simulink model "BEV_Laengsdynamikmodell_v2"  (R2023b)
settings: configuration reference "SharedConfig" (kept outside this file)
undefined symbols (not defined in the file): acc_cycle_flag, Analyse, battery, battery_builder_rtmsupport, config_battery, config_gearbox, config_Inverter, config_motor, config_vehicle, GB, gcbh, gearbox_map, k_FW, ModuleAssembly1, ModuleType1, motormap, motormap2
libraries: powerlib x37, nesl_utility x18, GD_Batterymodel_NSGAII_1_lib x12, BatteryProtection x9, fl_lib x7, dspstat3 x4, simulink x3, eePmsmCurrentReferenceGen x2, spsControlledCurrentSourceLib x2, spsVoltageMeasurementLib x2, batt_lib x1, BatteryBalancing x1
(part 5 of 6)

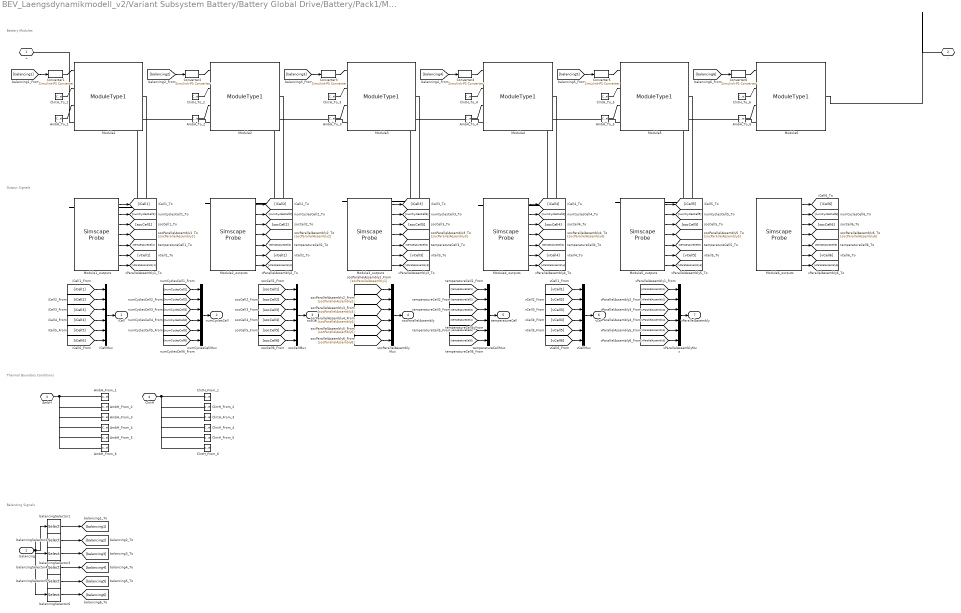
== system BEV_Laengsdynamikmodell_v2/Variant Subsystem Battery/Battery Global Drive/Battery/Pack1/ModuleAssembly2 ==
  note: Battery Modules
  note: Output Signals
  note: Thermal Boundary Conditions
  note: Balancing Signals
  balancing : Inport  PortDimensions=108
  AmbH_From_1 : ConnectionLabel  Label=ambH_1
  AmbH_From_2 : ConnectionLabel  Label=ambH_2
  AmbH_From_3 : ConnectionLabel  Label=ambH_3
  AmbH_From_4 : ConnectionLabel  Label=ambH_4
  AmbH_From_5 : ConnectionLabel  Label=ambH_5
  AmbH_From_6 : ConnectionLabel  Label=ambH_6
  AmbH_To_1 : ConnectionLabel  Label=ambH_1
  AmbH_To_2 : ConnectionLabel  Label=ambH_2
  AmbH_To_3 : ConnectionLabel  Label=ambH_3
  AmbH_To_4 : ConnectionLabel  Label=ambH_4
  AmbH_To_5 : ConnectionLabel  Label=ambH_5
  AmbH_To_6 : ConnectionLabel  Label=ambH_6
  ClntH_From_1 : ConnectionLabel  Label=clntH_1
  ClntH_From_2 : ConnectionLabel  Label=clntH_2
  ClntH_From_3 : ConnectionLabel  Label=clntH_3
  ClntH_From_4 : ConnectionLabel  Label=clntH_4
  ClntH_From_5 : ConnectionLabel  Label=clntH_5
  ClntH_From_6 : ConnectionLabel  Label=clntH_6
  ClntH_To_1 : ConnectionLabel  Label=clntH_1
  ClntH_To_2 : ConnectionLabel  Label=clntH_2
  ClntH_To_3 : ConnectionLabel  Label=clntH_3
  ClntH_To_4 : ConnectionLabel  Label=clntH_4
  ClntH_To_5 : ConnectionLabel  Label=clntH_5
  ClntH_To_6 : ConnectionLabel  Label=clntH_6
  Converter{1..6} (6 alike) : nesl_utility/Simulink-PS Converter  PhysicalDomain=network_engine_domain  SubClassName=ps_input  LeftPortType=input  RightPortType=output  PseudoPeriodic=off  Frequencies=[]  NoiseDistribution=none  NoiseParameters=[]  Unit=1  AffineConversion=off  FilteringAndDerivatives=provide  SimscapeFilterOrder=1  InputFilterTimeConstant=0.001  UdotUserProvided=0
  Module1 : GD_Batterymodel_NSGAII_1_lib/Modules/ModuleType1  SOC_vecCell=ModuleType1.SOC_vecCell  T_vecCell=ModuleType1.T_vecCell K  V0_matCell=ModuleType1.V0_matCell V  V_rangeCell=ModuleType1.V_rangeCell V  R0_matCell=ModuleType1.R0_matCell Ohm  AHCell=ModuleType1.AHCell A*hr  extrapolation_optionCell=simscape.enum.extrapolation.nearest  R1_matCell=ModuleType1.R1_matCell Ohm  tau1_matCell=ModuleType1.tau1_matCell s  R2_matCell=ModuleType1.R2_matCell Ohm  tau2_matCell=ModuleType1.tau2_matCell s  thermal_massCell=ModuleType1.thermal_massCell J/K  CoolantResistance=ModuleType1.CoolantResistance K/W  AmbientResistance=ModuleType1.AmbientResistance K/W  CellBalancingClosedResistance=ModuleType1.CellBalancingClosedResistance Ohm  CellBalancingOpenConductance=ModuleType1.CellBalancingOpenConductance 1/Ohm  CellBalancingThreshold=ModuleType1.CellBalancingThreshold  CellBalancingResistance=ModuleType1.CellBalancingResistance Ohm  P=1  S=18  iCell_specify=on  iCell_priority=None  iCell=ModuleAssembly2.Module1.iCell A  iCell_nominal_specify=off  iCell_nominal_unit=A  iCell_nominal_value=1  vCell_specify=on  vCell_priority=None  vCell=ModuleAssembly2.Module1.vCell V  vCell_nominal_specify=off  vCell_nominal_unit=V  vCell_nominal_value=1  socCell_specify=on  socCell_priority=High  socCell=ModuleAssembly2.Module1.socCell  socCell_nominal_specify=off  socCell_nominal_unit=1  socCell_nominal_value=1  numCyclesCell_specify=on  numCyclesCell_priority=High  numCyclesCell=ModuleAssembly2.Module1.numCyclesCell  numCyclesCell_nominal_specify=off  numCyclesCell_nominal_unit=1  numCyclesCell_nominal_value=1  temperatureCell_specify=on  temperatureCell_priority=High  temperatureCell=ModuleAssembly2.Module1.temperatureCell K  temperatureCell_nominal_specify=off  temperatureCell_nominal_unit=K  temperatureCell_nominal_value=1  vParallelAssembly_specify=on  vParallelAssembly_priority=None  vParallelAssembly=ModuleAssembly2.Module1.vParallelAssembly V  vParallelAssembly_nominal_specify=off  vParallelAssembly_nominal_unit=V  vParallelAssembly_nominal_value=1  socParallelAssembly_specify=on  socParallelAssembly_priority=None  socParallelAssembly=ModuleAssembly2.Module1.socParallelAssembly  socParallelAssembly_nominal_specify=off  socParallelAssembly_nominal_unit=1  socParallelAssembly_nominal_value=1
      settings: InternalSimscapePortConfiguration="{\"Bottom\":[{\"id\":\"n\",\"label\":\"-\",\"type\":\"foundation.electrical.electrical\"}],\"Left\":[{\"id\":\"enableCellBalancing\",\"label\":\"CB\",\"type\":\"input\"},{\"id\":\"ClntH\",\"label\":\"ClntH\",\"type\":\"foundation.thermal.thermal\"},{\"id\":\"AmbH\",\"label\":\"AmbH\",\"type\":\"foundation.thermal.thermal\"}],\"Right\":[],\"Top\":[{\"id\":\"p\",\"label\":\"+\",\"type\":\"foundation.electrical.electrical\"}]}"
  Module1_outputs : SimscapeProbe  BoundBlock=292794  Variables={iCell, numCyclesCell, socCell, socParallelAssembly, temperatureCell, vCell, vParallelAssembly}
  Module2 : GD_Batterymodel_NSGAII_1_lib/Modules/ModuleType1  SOC_vecCell=ModuleType1.SOC_vecCell  T_vecCell=ModuleType1.T_vecCell K  V0_matCell=ModuleType1.V0_matCell V  V_rangeCell=ModuleType1.V_rangeCell V  R0_matCell=ModuleType1.R0_matCell Ohm  AHCell=ModuleType1.AHCell A*hr  extrapolation_optionCell=simscape.enum.extrapolation.nearest  R1_matCell=ModuleType1.R1_matCell Ohm  tau1_matCell=ModuleType1.tau1_matCell s  R2_matCell=ModuleType1.R2_matCell Ohm  tau2_matCell=ModuleType1.tau2_matCell s  thermal_massCell=ModuleType1.thermal_massCell J/K  CoolantResistance=ModuleType1.CoolantResistance K/W  AmbientResistance=ModuleType1.AmbientResistance K/W  CellBalancingClosedResistance=ModuleType1.CellBalancingClosedResistance Ohm  CellBalancingOpenConductance=ModuleType1.CellBalancingOpenConductance 1/Ohm  CellBalancingThreshold=ModuleType1.CellBalancingThreshold  CellBalancingResistance=ModuleType1.CellBalancingResistance Ohm  P=1  S=18  iCell_specify=on  iCell_priority=None  iCell=ModuleAssembly2.Module2.iCell A  iCell_nominal_specify=off  iCell_nominal_unit=A  iCell_nominal_value=1  vCell_specify=on  vCell_priority=None  vCell=ModuleAssembly2.Module2.vCell V  vCell_nominal_specify=off  vCell_nominal_unit=V  vCell_nominal_value=1  socCell_specify=on  socCell_priority=High  socCell=ModuleAssembly2.Module2.socCell  socCell_nominal_specify=off  socCell_nominal_unit=1  socCell_nominal_value=1  numCyclesCell_specify=on  numCyclesCell_priority=High  numCyclesCell=ModuleAssembly2.Module2.numCyclesCell  numCyclesCell_nominal_specify=off  numCyclesCell_nominal_unit=1  numCyclesCell_nominal_value=1  temperatureCell_specify=on  temperatureCell_priority=High  temperatureCell=ModuleAssembly2.Module2.temperatureCell K  temperatureCell_nominal_specify=off  temperatureCell_nominal_unit=K  temperatureCell_nominal_value=1  vParallelAssembly_specify=on  vParallelAssembly_priority=None  vParallelAssembly=ModuleAssembly2.Module2.vParallelAssembly V  vParallelAssembly_nominal_specify=off  vParallelAssembly_nominal_unit=V  vParallelAssembly_nominal_value=1  socParallelAssembly_specify=on  socParallelAssembly_priority=None  socParallelAssembly=ModuleAssembly2.Module2.socParallelAssembly  socParallelAssembly_nominal_specify=off  socParallelAssembly_nominal_unit=1  socParallelAssembly_nominal_value=1
      settings: InternalSimscapePortConfiguration="{\"Bottom\":[{\"id\":\"n\",\"label\":\"-\",\"type\":\"foundation.electrical.electrical\"}],\"Left\":[{\"id\":\"enableCellBalancing\",\"label\":\"CB\",\"type\":\"input\"},{\"id\":\"ClntH\",\"label\":\"ClntH\",\"type\":\"foundation.thermal.thermal\"},{\"id\":\"AmbH\",\"label\":\"AmbH\",\"type\":\"foundation.thermal.thermal\"}],\"Right\":[],\"Top\":[{\"id\":\"p\",\"label\":\"+\",\"type\":\"foundation.electrical.electrical\"}]}"
  Module2_outputs : SimscapeProbe  BoundBlock=292796  Variables={iCell, numCyclesCell, socCell, socParallelAssembly, temperatureCell, vCell, vParallelAssembly}
  Module3 : GD_Batterymodel_NSGAII_1_lib/Modules/ModuleType1  SOC_vecCell=ModuleType1.SOC_vecCell  T_vecCell=ModuleType1.T_vecCell K  V0_matCell=ModuleType1.V0_matCell V  V_rangeCell=ModuleType1.V_rangeCell V  R0_matCell=ModuleType1.R0_matCell Ohm  AHCell=ModuleType1.AHCell A*hr  extrapolation_optionCell=simscape.enum.extrapolation.nearest  R1_matCell=ModuleType1.R1_matCell Ohm  tau1_matCell=ModuleType1.tau1_matCell s  R2_matCell=ModuleType1.R2_matCell Ohm  tau2_matCell=ModuleType1.tau2_matCell s  thermal_massCell=ModuleType1.thermal_massCell J/K  CoolantResistance=ModuleType1.CoolantResistance K/W  AmbientResistance=ModuleType1.AmbientResistance K/W  CellBalancingClosedResistance=ModuleType1.CellBalancingClosedResistance Ohm  CellBalancingOpenConductance=ModuleType1.CellBalancingOpenConductance 1/Ohm  CellBalancingThreshold=ModuleType1.CellBalancingThreshold  CellBalancingResistance=ModuleType1.CellBalancingResistance Ohm  P=1  S=18  iCell_specify=on  iCell_priority=None  iCell=ModuleAssembly2.Module3.iCell A  iCell_nominal_specify=off  iCell_nominal_unit=A  iCell_nominal_value=1  vCell_specify=on  vCell_priority=None  vCell=ModuleAssembly2.Module3.vCell V  vCell_nominal_specify=off  vCell_nominal_unit=V  vCell_nominal_value=1  socCell_specify=on  socCell_priority=High  socCell=ModuleAssembly2.Module3.socCell  socCell_nominal_specify=off  socCell_nominal_unit=1  socCell_nominal_value=1  numCyclesCell_specify=on  numCyclesCell_priority=High  numCyclesCell=ModuleAssembly2.Module3.numCyclesCell  numCyclesCell_nominal_specify=off  numCyclesCell_nominal_unit=1  numCyclesCell_nominal_value=1  temperatureCell_specify=on  temperatureCell_priority=High  temperatureCell=ModuleAssembly2.Module3.temperatureCell K  temperatureCell_nominal_specify=off  temperatureCell_nominal_unit=K  temperatureCell_nominal_value=1  vParallelAssembly_specify=on  vParallelAssembly_priority=None  vParallelAssembly=ModuleAssembly2.Module3.vParallelAssembly V  vParallelAssembly_nominal_specify=off  vParallelAssembly_nominal_unit=V  vParallelAssembly_nominal_value=1  socParallelAssembly_specify=on  socParallelAssembly_priority=None  socParallelAssembly=ModuleAssembly2.Module3.socParallelAssembly  socParallelAssembly_nominal_specify=off  socParallelAssembly_nominal_unit=1  socParallelAssembly_nominal_value=1
      settings: InternalSimscapePortConfiguration="{\"Bottom\":[{\"id\":\"n\",\"label\":\"-\",\"type\":\"foundation.electrical.electrical\"}],\"Left\":[{\"id\":\"enableCellBalancing\",\"label\":\"CB\",\"type\":\"input\"},{\"id\":\"ClntH\",\"label\":\"ClntH\",\"type\":\"foundation.thermal.thermal\"},{\"id\":\"AmbH\",\"label\":\"AmbH\",\"type\":\"foundation.thermal.thermal\"}],\"Right\":[],\"Top\":[{\"id\":\"p\",\"label\":\"+\",\"type\":\"foundation.electrical.electrical\"}]}"
  Module3_outputs : SimscapeProbe  BoundBlock=292798  Variables={iCell, numCyclesCell, socCell, socParallelAssembly, temperatureCell, vCell, vParallelAssembly}
  Module4 : GD_Batterymodel_NSGAII_1_lib/Modules/ModuleType1  SOC_vecCell=ModuleType1.SOC_vecCell  T_vecCell=ModuleType1.T_vecCell K  V0_matCell=ModuleType1.V0_matCell V  V_rangeCell=ModuleType1.V_rangeCell V  R0_matCell=ModuleType1.R0_matCell Ohm  AHCell=ModuleType1.AHCell A*hr  extrapolation_optionCell=simscape.enum.extrapolation.nearest  R1_matCell=ModuleType1.R1_matCell Ohm  tau1_matCell=ModuleType1.tau1_matCell s  R2_matCell=ModuleType1.R2_matCell Ohm  tau2_matCell=ModuleType1.tau2_matCell s  thermal_massCell=ModuleType1.thermal_massCell J/K  CoolantResistance=ModuleType1.CoolantResistance K/W  AmbientResistance=ModuleType1.AmbientResistance K/W  CellBalancingClosedResistance=ModuleType1.CellBalancingClosedResistance Ohm  CellBalancingOpenConductance=ModuleType1.CellBalancingOpenConductance 1/Ohm  CellBalancingThreshold=ModuleType1.CellBalancingThreshold  CellBalancingResistance=ModuleType1.CellBalancingResistance Ohm  P=1  S=18  iCell_specify=on  iCell_priority=None  iCell=ModuleAssembly2.Module4.iCell A  iCell_nominal_specify=off  iCell_nominal_unit=A  iCell_nominal_value=1  vCell_specify=on  vCell_priority=None  vCell=ModuleAssembly2.Module4.vCell V  vCell_nominal_specify=off  vCell_nominal_unit=V  vCell_nominal_value=1  socCell_specify=on  socCell_priority=High  socCell=ModuleAssembly2.Module4.socCell  socCell_nominal_specify=off  socCell_nominal_unit=1  socCell_nominal_value=1  numCyclesCell_specify=on  numCyclesCell_priority=High  numCyclesCell=ModuleAssembly2.Module4.numCyclesCell  numCyclesCell_nominal_specify=off  numCyclesCell_nominal_unit=1  numCyclesCell_nominal_value=1  temperatureCell_specify=on  temperatureCell_priority=High  temperatureCell=ModuleAssembly2.Module4.temperatureCell K  temperatureCell_nominal_specify=off  temperatureCell_nominal_unit=K  temperatureCell_nominal_value=1  vParallelAssembly_specify=on  vParallelAssembly_priority=None  vParallelAssembly=ModuleAssembly2.Module4.vParallelAssembly V  vParallelAssembly_nominal_specify=off  vParallelAssembly_nominal_unit=V  vParallelAssembly_nominal_value=1  socParallelAssembly_specify=on  socParallelAssembly_priority=None  socParallelAssembly=ModuleAssembly2.Module4.socParallelAssembly  socParallelAssembly_nominal_specify=off  socParallelAssembly_nominal_unit=1  socParallelAssembly_nominal_value=1
      settings: InternalSimscapePortConfiguration="{\"Bottom\":[{\"id\":\"n\",\"label\":\"-\",\"type\":\"foundation.electrical.electrical\"}],\"Left\":[{\"id\":\"enableCellBalancing\",\"label\":\"CB\",\"type\":\"input\"},{\"id\":\"ClntH\",\"label\":\"ClntH\",\"type\":\"foundation.thermal.thermal\"},{\"id\":\"AmbH\",\"label\":\"AmbH\",\"type\":\"foundation.thermal.thermal\"}],\"Right\":[],\"Top\":[{\"id\":\"p\",\"label\":\"+\",\"type\":\"foundation.electrical.electrical\"}]}"
  Module4_outputs : SimscapeProbe  BoundBlock=292800  Variables={iCell, numCyclesCell, socCell, socParallelAssembly, temperatureCell, vCell, vParallelAssembly}
  Module5 : GD_Batterymodel_NSGAII_1_lib/Modules/ModuleType1  SOC_vecCell=ModuleType1.SOC_vecCell  T_vecCell=ModuleType1.T_vecCell K  V0_matCell=ModuleType1.V0_matCell V  V_rangeCell=ModuleType1.V_rangeCell V  R0_matCell=ModuleType1.R0_matCell Ohm  AHCell=ModuleType1.AHCell A*hr  extrapolation_optionCell=simscape.enum.extrapolation.nearest  R1_matCell=ModuleType1.R1_matCell Ohm  tau1_matCell=ModuleType1.tau1_matCell s  R2_matCell=ModuleType1.R2_matCell Ohm  tau2_matCell=ModuleType1.tau2_matCell s  thermal_massCell=ModuleType1.thermal_massCell J/K  CoolantResistance=ModuleType1.CoolantResistance K/W  AmbientResistance=ModuleType1.AmbientResistance K/W  CellBalancingClosedResistance=ModuleType1.CellBalancingClosedResistance Ohm  CellBalancingOpenConductance=ModuleType1.CellBalancingOpenConductance 1/Ohm  CellBalancingThreshold=ModuleType1.CellBalancingThreshold  CellBalancingResistance=ModuleType1.CellBalancingResistance Ohm  P=1  S=18  iCell_specify=on  iCell_priority=None  iCell=ModuleAssembly2.Module5.iCell A  iCell_nominal_specify=off  iCell_nominal_unit=A  iCell_nominal_value=1  vCell_specify=on  vCell_priority=None  vCell=ModuleAssembly2.Module5.vCell V  vCell_nominal_specify=off  vCell_nominal_unit=V  vCell_nominal_value=1  socCell_specify=on  socCell_priority=High  socCell=ModuleAssembly2.Module5.socCell  socCell_nominal_specify=off  socCell_nominal_unit=1  socCell_nominal_value=1  numCyclesCell_specify=on  numCyclesCell_priority=High  numCyclesCell=ModuleAssembly2.Module5.numCyclesCell  numCyclesCell_nominal_specify=off  numCyclesCell_nominal_unit=1  numCyclesCell_nominal_value=1  temperatureCell_specify=on  temperatureCell_priority=High  temperatureCell=ModuleAssembly2.Module5.temperatureCell K  temperatureCell_nominal_specify=off  temperatureCell_nominal_unit=K  temperatureCell_nominal_value=1  vParallelAssembly_specify=on  vParallelAssembly_priority=None  vParallelAssembly=ModuleAssembly2.Module5.vParallelAssembly V  vParallelAssembly_nominal_specify=off  vParallelAssembly_nominal_unit=V  vParallelAssembly_nominal_value=1  socParallelAssembly_specify=on  socParallelAssembly_priority=None  socParallelAssembly=ModuleAssembly2.Module5.socParallelAssembly  socParallelAssembly_nominal_specify=off  socParallelAssembly_nominal_unit=1  socParallelAssembly_nominal_value=1
      settings: InternalSimscapePortConfiguration="{\"Bottom\":[{\"id\":\"n\",\"label\":\"-\",\"type\":\"foundation.electrical.electrical\"}],\"Left\":[{\"id\":\"enableCellBalancing\",\"label\":\"CB\",\"type\":\"input\"},{\"id\":\"ClntH\",\"label\":\"ClntH\",\"type\":\"foundation.thermal.thermal\"},{\"id\":\"AmbH\",\"label\":\"AmbH\",\"type\":\"foundation.thermal.thermal\"}],\"Right\":[],\"Top\":[{\"id\":\"p\",\"label\":\"+\",\"type\":\"foundation.electrical.electrical\"}]}"
  Module5_outputs : SimscapeProbe  BoundBlock=292802  Variables={iCell, numCyclesCell, socCell, socParallelAssembly, temperatureCell, vCell, vParallelAssembly}
  Module6 : GD_Batterymodel_NSGAII_1_lib/Modules/ModuleType1  SOC_vecCell=ModuleType1.SOC_vecCell  T_vecCell=ModuleType1.T_vecCell K  V0_matCell=ModuleType1.V0_matCell V  V_rangeCell=ModuleType1.V_rangeCell V  R0_matCell=ModuleType1.R0_matCell Ohm  AHCell=ModuleType1.AHCell A*hr  extrapolation_optionCell=simscape.enum.extrapolation.nearest  R1_matCell=ModuleType1.R1_matCell Ohm  tau1_matCell=ModuleType1.tau1_matCell s  R2_matCell=ModuleType1.R2_matCell Ohm  tau2_matCell=ModuleType1.tau2_matCell s  thermal_massCell=ModuleType1.thermal_massCell J/K  CoolantResistance=ModuleType1.CoolantResistance K/W  AmbientResistance=ModuleType1.AmbientResistance K/W  CellBalancingClosedResistance=ModuleType1.CellBalancingClosedResistance Ohm  CellBalancingOpenConductance=ModuleType1.CellBalancingOpenConductance 1/Ohm  CellBalancingThreshold=ModuleType1.CellBalancingThreshold  CellBalancingResistance=ModuleType1.CellBalancingResistance Ohm  P=1  S=18  iCell_specify=on  iCell_priority=None  iCell=ModuleAssembly2.Module6.iCell A  iCell_nominal_specify=off  iCell_nominal_unit=A  iCell_nominal_value=1  vCell_specify=on  vCell_priority=None  vCell=ModuleAssembly2.Module6.vCell V  vCell_nominal_specify=off  vCell_nominal_unit=V  vCell_nominal_value=1  socCell_specify=on  socCell_priority=High  socCell=ModuleAssembly2.Module6.socCell  socCell_nominal_specify=off  socCell_nominal_unit=1  socCell_nominal_value=1  numCyclesCell_specify=on  numCyclesCell_priority=High  numCyclesCell=ModuleAssembly2.Module6.numCyclesCell  numCyclesCell_nominal_specify=off  numCyclesCell_nominal_unit=1  numCyclesCell_nominal_value=1  temperatureCell_specify=on  temperatureCell_priority=High  temperatureCell=ModuleAssembly2.Module6.temperatureCell K  temperatureCell_nominal_specify=off  temperatureCell_nominal_unit=K  temperatureCell_nominal_value=1  vParallelAssembly_specify=on  vParallelAssembly_priority=None  vParallelAssembly=ModuleAssembly2.Module6.vParallelAssembly V  vParallelAssembly_nominal_specify=off  vParallelAssembly_nominal_unit=V  vParallelAssembly_nominal_value=1  socParallelAssembly_specify=on  socParallelAssembly_priority=None  socParallelAssembly=ModuleAssembly2.Module6.socParallelAssembly  socParallelAssembly_nominal_specify=off  socParallelAssembly_nominal_unit=1  socParallelAssembly_nominal_value=1
      settings: InternalSimscapePortConfiguration="{\"Bottom\":[{\"id\":\"n\",\"label\":\"-\",\"type\":\"foundation.electrical.electrical\"}],\"Left\":[{\"id\":\"enableCellBalancing\",\"label\":\"CB\",\"type\":\"input\"},{\"id\":\"ClntH\",\"label\":\"ClntH\",\"type\":\"foundation.thermal.thermal\"},{\"id\":\"AmbH\",\"label\":\"AmbH\",\"type\":\"foundation.thermal.thermal\"}],\"Right\":[],\"Top\":[{\"id\":\"p\",\"label\":\"+\",\"type\":\"foundation.electrical.electrical\"}]}"
  Module6_outputs : SimscapeProbe  BoundBlock=292804  Variables={iCell, numCyclesCell, socCell, socParallelAssembly, temperatureCell, vCell, vParallelAssembly}
  balancingSelector1 : Selector  InputPortWidth=108  IndexOptions=Index vector (dialog)  Indices="[1   2   3   4   5   6   7   8   9  10  11  12  13  14  15  16  17  18]"  OutputSizes=1
  balancingSelector2 : Selector  InputPortWidth=108  IndexOptions=Index vector (dialog)  Indices="[19  20  21  22  23  24  25  26  27  28  29  30  31  32  33  34  35  36]"  OutputSizes=1
  balancingSelector3 : Selector  InputPortWidth=108  IndexOptions=Index vector (dialog)  Indices="[37  38  39  40  41  42  43  44  45  46  47  48  49  50  51  52  53  54]"  OutputSizes=1
  balancingSelector4 : Selector  InputPortWidth=108  IndexOptions=Index vector (dialog)  Indices="[55  56  57  58  59  60  61  62  63  64  65  66  67  68  69  70  71  72]"  OutputSizes=1
  balancingSelector5 : Selector  InputPortWidth=108  IndexOptions=Index vector (dialog)  Indices="[73  74  75  76  77  78  79  80  81  82  83  84  85  86  87  88  89  90]"  OutputSizes=1
  balancingSelector6 : Selector  InputPortWidth=108  IndexOptions=Index vector (dialog)  Indices="[91   92   93   94   95   96   97   98   99  100  101  102  103  104  105  106  107  108]"  OutputSizes=1
  iCellMux : Mux  Inputs=6
  numCyclesCellMux : Mux  Inputs=6
  socCellMux : Mux  Inputs=6
  socParallelAssemblyMux : Mux  Inputs=6
  temperatureCellMux : Mux  Inputs=6
  vCellMux : Mux  Inputs=6
  vParallelAssemblyMux : Mux  Inputs=6
  + : PMIOPort  Side=Left
  - : PMIOPort  Port=2  Side=Right
  AmbH : PMIOPort  Port=3  Side=Right  ConnectionType=Connection: foundation.thermal.thermal
  ClntH : PMIOPort  Port=4  Side=Right  ConnectionType=Connection: foundation.thermal.thermal
  iCell : Outport
  numCyclesCell : Outport  Port=2
  socCell : Outport  Port=3
  socParallelAssembly : Outport  Port=4
  temperatureCell : Outport  Port=5
  vCell : Outport  Port=6
  vParallelAssembly : Outport  Port=7
  wires:
  Module1_outputs/1 -> [iCell1]
  iCellMux/1 -> iCell/1
  [iCell1] -> iCellMux/1
  Module1_outputs/2 -> [numCyclesCell1]
  numCyclesCellMux/1 -> numCyclesCell/1
  [numCyclesCell1] -> numCyclesCellMux/1
  Module1_outputs/3 -> [socCell1]
  socCellMux/1 -> socCell/1
  [socCell1] -> socCellMux/1
  Module1_outputs/4 -> [socParallelAssembly1]
  socParallelAssemblyMux/1 -> socParallelAssembly/1
  [socParallelAssembly1] -> socParallelAssemblyMux/1
  Module1_outputs/5 -> [temperatureCell1]
  temperatureCellMux/1 -> temperatureCell/1
  [temperatureCell1] -> temperatureCellMux/1
  Module1_outputs/6 -> [vCell1]
  vCellMux/1 -> vCell/1
  [vCell1] -> vCellMux/1
  Module1_outputs/7 -> [vParallelAssembly1]
  vParallelAssemblyMux/1 -> vParallelAssembly/1
  [vParallelAssembly1] -> vParallelAssemblyMux/1
  Module2_outputs/1 -> [iCell2]
  [iCell2] -> iCellMux/2
  Module2_outputs/2 -> [numCyclesCell2]
  [numCyclesCell2] -> numCyclesCellMux/2
  Module2_outputs/3 -> [socCell2]
  [socCell2] -> socCellMux/2
  Module2_outputs/4 -> [socParallelAssembly2]
  [socParallelAssembly2] -> socParallelAssemblyMux/2
  Module2_outputs/5 -> [temperatureCell2]
  [temperatureCell2] -> temperatureCellMux/2
  Module2_outputs/6 -> [vCell2]
  [vCell2] -> vCellMux/2
  Module2_outputs/7 -> [vParallelAssembly2]
  [vParallelAssembly2] -> vParallelAssemblyMux/2
  Module3_outputs/1 -> [iCell3]
  [iCell3] -> iCellMux/3
  Module3_outputs/2 -> [numCyclesCell3]
  [numCyclesCell3] -> numCyclesCellMux/3
  Module3_outputs/3 -> [socCell3]
  [socCell3] -> socCellMux/3
  Module3_outputs/4 -> [socParallelAssembly3]
  [socParallelAssembly3] -> socParallelAssemblyMux/3
  Module3_outputs/5 -> [temperatureCell3]
  [temperatureCell3] -> temperatureCellMux/3
  Module3_outputs/6 -> [vCell3]
  [vCell3] -> vCellMux/3
  Module3_outputs/7 -> [vParallelAssembly3]
  [vParallelAssembly3] -> vParallelAssemblyMux/3
  Module4_outputs/1 -> [iCell4]
  [iCell4] -> iCellMux/4
  Module4_outputs/2 -> [numCyclesCell4]
  [numCyclesCell4] -> numCyclesCellMux/4
  Module4_outputs/3 -> [socCell4]
  [socCell4] -> socCellMux/4
  Module4_outputs/4 -> [socParallelAssembly4]
  [socParallelAssembly4] -> socParallelAssemblyMux/4
  Module4_outputs/5 -> [temperatureCell4]
  [temperatureCell4] -> temperatureCellMux/4
  Module4_outputs/6 -> [vCell4]
  [vCell4] -> vCellMux/4
  Module4_outputs/7 -> [vParallelAssembly4]
  [vParallelAssembly4] -> vParallelAssemblyMux/4
  Module5_outputs/1 -> [iCell5]
  [iCell5] -> iCellMux/5
  Module5_outputs/2 -> [numCyclesCell5]
  [numCyclesCell5] -> numCyclesCellMux/5
  Module5_outputs/3 -> [socCell5]
  [socCell5] -> socCellMux/5
  Module5_outputs/4 -> [socParallelAssembly5]
  [socParallelAssembly5] -> socParallelAssemblyMux/5
  Module5_outputs/5 -> [temperatureCell5]
  [temperatureCell5] -> temperatureCellMux/5
  Module5_outputs/6 -> [vCell5]
  [vCell5] -> vCellMux/5
  Module5_outputs/7 -> [vParallelAssembly5]
  [vParallelAssembly5] -> vParallelAssemblyMux/5
  Module6_outputs/1 -> [iCell6]
  [iCell6] -> iCellMux/6
  Module6_outputs/2 -> [numCyclesCell6]
  [numCyclesCell6] -> numCyclesCellMux/6
  Module6_outputs/3 -> [socCell6]
  [socCell6] -> socCellMux/6
  Module6_outputs/4 -> [socParallelAssembly6]
  [socParallelAssembly6] -> socParallelAssemblyMux/6
  Module6_outputs/5 -> [temperatureCell6]
  [temperatureCell6] -> temperatureCellMux/6
  Module6_outputs/6 -> [vCell6]
  [vCell6] -> vCellMux/6
  Module6_outputs/7 -> [vParallelAssembly6]
  [vParallelAssembly6] -> vParallelAssemblyMux/6
  [balancing1] -> Converter1/1
  balancing/1 -> balancingSelector1/1, balancingSelector2/1, balancingSelector3/1, balancingSelector4/1, balancingSelector5/1, balancingSelector6/1
  balancingSelector1/1 -> [balancing1]
  [balancing2] -> Converter2/1
  balancingSelector2/1 -> [balancing2]
  [balancing3] -> Converter3/1
  balancingSelector3/1 -> [balancing3]
  [balancing4] -> Converter4/1
  balancingSelector4/1 -> [balancing4]
  [balancing5] -> Converter5/1
  balancingSelector5/1 -> [balancing5]
  [balancing6] -> Converter6/1
  balancingSelector6/1 -> [balancing6]
  connections:
  Module2/LConn4 -- Module1/RConn1
  Module3/LConn4 -- Module2/RConn1
  Module4/LConn4 -- Module3/RConn1
  Module5/LConn4 -- Module4/RConn1
  Module6/LConn4 -- Module5/RConn1
  Module1/LConn4 -- +/RConn1
  Module6/RConn1 -- -/RConn1
  AmbH_To_1/LConn1 -- Module1/LConn3
  AmbH_From_1/LConn1 -- AmbH_From_2/LConn1 -- AmbH_From_3/LConn1 -- AmbH_From_4/LConn1 -- AmbH_From_5/LConn1 -- AmbH/RConn1 -- AmbH_From_6/LConn1
  AmbH_To_2/LConn1 -- Module2/LConn3
  AmbH_To_3/LConn1 -- Module3/LConn3
  AmbH_To_4/LConn1 -- Module4/LConn3
  AmbH_To_5/LConn1 -- Module5/LConn3
  AmbH_To_6/LConn1 -- Module6/LConn3
  ClntH_To_1/LConn1 -- Module1/LConn2
  ClntH_From_1/LConn1 -- ClntH_From_2/LConn1 -- ClntH_From_3/LConn1 -- ClntH_From_4/LConn1 -- ClntH_From_5/LConn1 -- ClntH/RConn1 -- ClntH_From_6/LConn1
  ClntH_To_2/LConn1 -- Module2/LConn2
  ClntH_To_3/LConn1 -- Module3/LConn2
  ClntH_To_4/LConn1 -- Module4/LConn2
  ClntH_To_5/LConn1 -- Module5/LConn2
  ClntH_To_6/LConn1 -- Module6/LConn2
  Converter1/RConn1 -- Module1/LConn1
  Converter2/RConn1 -- Module2/LConn1
  Converter3/RConn1 -- Module3/LConn1
  Converter4/RConn1 -- Module4/LConn1
  Converter5/RConn1 -- Module5/LConn1
  Converter6/RConn1 -- Module6/LConn1

== system BEV_Laengsdynamikmodell_v2/Variant Subsystem Gearbox/Gearbox Analytic/Variant Subsystem Analytic GB/Einstufig_Achsparallel/Ölpumpe ==
  nrad : Inport
  Constant : Constant  Value=config_gearbox.power_oilpump
  Constant1 : Constant  Value=1.5e3
  Product : Product  Inputs=*/*
  Scope : Scope
  power_oilpump : Outport
  wires:
  Product/1 -> power_oilpump/1, Scope/1
  Constant1/1 -> Product/2
  nrad/1 -> Product/1
  Constant/1 -> Product/3

== system BEV_Laengsdynamikmodell_v2/Variant Subsystem Gearbox/Gearbox Analytic/Variant Subsystem Analytic GB/Zweistufig_Achsparallel/Ölpumpe ==
  nrad : Inport
  Constant : Constant  Value=config_gearbox.power_oilpump
  Constant1 : Constant  Value=15e3
  Product : Product  Inputs=*/*
  Scope : Scope
  power_oilpump : Outport
  wires:
  Product/1 -> power_oilpump/1, Scope/1
  Constant1/1 -> Product/2
  nrad/1 -> Product/1
  Constant/1 -> Product/3

== system BEV_Laengsdynamikmodell_v2/Variant Subsystem Gearbox/Gearbox Analytic/Variant Subsystem Analytic GB/Zweistufig_Koaxial/Ölpumpe ==
  nrad : Inport
  Constant : Constant  Value=config_gearbox.power_oilpump
  Constant1 : Constant  Value=1.5e3
  Product : Product  Inputs=*/*
  Scope : Scope
  power_oilpump : Outport
  wires:
  Product/1 -> power_oilpump/1, Scope/1
  Constant1/1 -> Product/2
  nrad/1 -> Product/1
  Constant/1 -> Product/3

== system BEV_Laengsdynamikmodell_v2/Variant Subsystem Gearbox/Gearbox Lookup-Table/Variant Subsystem/ETA_map/Lookup Gearbox ==
  note: 1) Add Subsystem or Model blocks as valid variant choices.
      | 2) You cannot connect blocks at this level. At simulation, connectivity is automatically
      | determined, based on the active variant and port name matching.
  Torque : Inport
  RPM : Inport  Port=2
  Temp : Inport  Port=3
  Lookup with Temp : Subsystem  VariantControl=gearbox_map.dim_lookup == 3
  Lookup without Temp : Subsystem  VariantControl=gearbox_map.dim_lookup == 2
  Eta : Outport

== system BEV_Laengsdynamikmodell_v2/Variant Subsystem Gearbox/Gearbox Lookup-Table/Variant Subsystem/ETA_map/Oilpump ==
  rpm_wheel : Inport
  Constant7 : Constant  Value=config_gearbox.power_oilpump
  Constant8 : Constant  Value=1.5e3
  Product4 : Product  Inputs=**/
  loss_oilpump : Outport
  wires:
  rpm_wheel/1 -> Product4/1
  Constant8/1 -> Product4/3
  Constant7/1 -> Product4/2
  Product4/1 -> loss_oilpump/1  "loss_oilpump"

== system BEV_Laengsdynamikmodell_v2/Variant Subsystem Gearbox/Gearbox Lookup-Table/Variant Subsystem/LOSS_map/Lookup Gearbox ==
  note: 1) Add Subsystem or Model blocks as valid variant choices.
      | 2) You cannot connect blocks at this level. At simulation, connectivity is automatically
      | determined, based on the active variant and port name matching.
  Torque : Inport
  RPM : Inport  Port=2
  Temp : Inport  Port=3
  Lookup with Temp : Subsystem  VariantControl=gearbox_map.dim_lookup == 3
  Lookup without Temp : Subsystem  VariantControl=gearbox_map.dim_lookup == 2
  Loss : Outport

== system BEV_Laengsdynamikmodell_v2/Variant Subsystem Gearbox/Gearbox Lookup-Table/Variant Subsystem/LOSS_map/Oilpump ==
  rpm_wheel : Inport
  Constant7 : Constant  Value=config_gearbox.power_oilpump
  Constant8 : Constant  Value=1.5e3
  Product4 : Product  Inputs=**/
  loss_oilpump : Outport
  wires:
  Product4/1 -> loss_oilpump/1  "loss_oilpump"
  Constant7/1 -> Product4/2
  Constant8/1 -> Product4/3
  rpm_wheel/1 -> Product4/1

== system BEV_Laengsdynamikmodell_v2/Variant Subsystem Gearbox/Gearbox Lookup-Table/Variant Subsystem/ETA_map/Lookup Gearbox/Lookup with Temp ==
  Torque : Inport
  RPM : Inport  Port=2
  Temp : Inport  Port=3
  n-D Lookup Table : Lookup_n-D  NumberOfTableDimensions=3  BreakpointsForDimension1=gearbox_map.torque  BreakpointsForDimension2=gearbox_map.rpm  BreakpointsForDimension3=gearbox_map.temperature  Table=gearbox_map.eta  UseLastTableValue=on  InternalRulePriority=Speed  RndMeth=Simplest
      settings: InputPortMap=u0,u1,u2
  Eta : Outport
  wires:
  Torque/1 -> n-D Lookup Table/1
  RPM/1 -> n-D Lookup Table/2
  Temp/1 -> n-D Lookup Table/3
  n-D Lookup Table/1 -> Eta/1

== system BEV_Laengsdynamikmodell_v2/Variant Subsystem Gearbox/Gearbox Lookup-Table/Variant Subsystem/ETA_map/Lookup Gearbox/Lookup without Temp ==
  Torque : Inport
  RPM : Inport  Port=2
  n-D Lookup Table : Lookup_n-D  BreakpointsForDimension1=gearbox_map.torque  BreakpointsForDimension2=gearbox_map.rpm  BreakpointsForDimension3=gearbox_map.temperature  Table=gearbox_map.eta  UseLastTableValue=on  InternalRulePriority=Speed  RndMeth=Simplest
      settings: InputPortMap=u0,u1
  Eta : Outport
  wires:
  Torque/1 -> n-D Lookup Table/1
  RPM/1 -> n-D Lookup Table/2
  n-D Lookup Table/1 -> Eta/1

== system BEV_Laengsdynamikmodell_v2/Variant Subsystem Gearbox/Gearbox Lookup-Table/Variant Subsystem/LOSS_map/Lookup Gearbox/Lookup with Temp ==
  Torque : Inport
  RPM : Inport  Port=2
  Temp : Inport  Port=3
  n-D Lookup Table : Lookup_n-D  NumberOfTableDimensions=3  BreakpointsForDimension1=gearbox_map.torque  BreakpointsForDimension2=gearbox_map.rpm  BreakpointsForDimension3=gearbox_map.temperature  Table=gearbox_map.loss  UseLastTableValue=on  InternalRulePriority=Speed  RndMeth=Simplest
      settings: InputPortMap=u0,u1,u2
  Loss : Outport
  wires:
  n-D Lookup Table/1 -> Loss/1
  Temp/1 -> n-D Lookup Table/3
  RPM/1 -> n-D Lookup Table/2
  Torque/1 -> n-D Lookup Table/1

== system BEV_Laengsdynamikmodell_v2/Variant Subsystem Gearbox/Gearbox Lookup-Table/Variant Subsystem/LOSS_map/Lookup Gearbox/Lookup without Temp ==
  Torque : Inport
  RPM : Inport  Port=2
  n-D Lookup Table : Lookup_n-D  BreakpointsForDimension1=gearbox_map.torque  BreakpointsForDimension2=gearbox_map.rpm  BreakpointsForDimension3=gearbox_map.temperature  Table=gearbox_map.loss  UseLastTableValue=on  InternalRulePriority=Speed  RndMeth=Simplest
      settings: InputPortMap=u0,u1
  Loss : Outport
  wires:
  n-D Lookup Table/1 -> Loss/1
  RPM/1 -> n-D Lookup Table/2
  Torque/1 -> n-D Lookup Table/1

== matlab function BEV_Laengsdynamikmodell_v2/Variant Subsystem Battery/Battery Analytic (RC3)/Battery/MATLAB Function1 ==
  data: u input; y output
function y = fcn(u)
if u == 1
    warning("Battery: LE drew more current then allowed")
end
y = u;

== matlab function BEV_Laengsdynamikmodell_v2/Variant Subsystem Inverter/Inverter Analytic/Variant Subsystem/IM_Inverter_IGBT_Analytic/Change parameters from datasheet here ==
  data: ic input; udc input; up input; fs input; CPloss_igbt output; CPloss_diode output; costheta input; Eon_igbt_nom input; Eoff_igbt_nom input; Erec_diode_nom input; SPloss_igbt output; SPloss_diode output; T_igbt input; T_diode input
function [CPloss_igbt,CPloss_diode,SPloss_igbt,SPloss_diode] = IGBT(ic,udc,up,fs,costheta,Eon_igbt_nom, Eoff_igbt_nom, Erec_diode_nom, T_igbt, T_diode)
%%%%%%%%%%%%%%%%%%%%%%%%%%% parameter table %%%%%%%%%%%%%%%%%%%%%%%%%%%%%%%
%%%%%%%%%%%%%%%%%%%%%%%%%%% varialbe table %%%%%%%%%%%%%%%%%%%%%%%%%%%%%%%%
% variavle name      meaning,                                                        unit
% ic,                operation current peak                                          (A)
% up,                operation voltage peak                                          (V)
% udc,               DC bus voltage,                                                 (V)
% fs,                switching frequency,                                            (Hz)
% costheta,          power factor,                                                   (none)
% CPloss_igbt,       conduction loss on IGBT,                                        (W)
% CPloss_diode,      conduction loss on the reverse paralleled diode,                (W)
% SPloss_igbt,       switching loss on IGBT,                                         (W)
% SPloss_diode,      switching loss on the reverse paralleled diode,                 (W)
%%%%%%%%%%%%%%%%%%%%%%%%%%%%%%%%%%%%%%%%%%%%%%%%%%%%%%%%%%%%%%%%%%%%%%%%%%%
parallel = 1;

ic = ic/parallel;

icn = 450;
uce_test = 400;
ifn = 450;
uf_test = 400;

T25 = 25;
T175 = 175;
uce0 = 0.75;
rc25 = 0.0005;
rc175 = 0.00089;
kCE = (rc175-rc25)/(T175-T25);
ud0 = 0.95;
rd25 = 0.00067;
rd175 = 0.00075;
kD = (rd175-rd25)/(T175-T25);
%%
rc = rc25 + (T_igbt - 25)*kCE;  
rd = rd25 + (T_diode - 25)*kD; 
uce = uce0 + ic*rc;             
uf = ud0 + ic*rd;            

m = up*sqrt(2)*2/udc; 

Eon_igbt = Eon_igbt_nom * ic/icn * udc/uce_test;    
Eoff_igbt = Eoff_igbt_nom * ic/ifn * udc/uce_test;         
Erec_diode = Erec_diode_nom * ic/ifn * udc/uf_test; 

CPloss_igbt = sqrt(2)*uce*ic*(1/2/pi+m*costheta/8) + 2*rc*ic*ic*(1/8+m*costheta/3/pi);
CPloss_diode = sqrt(2)*uf*ic*(1/2/pi-m*costheta/8) + 2*rd*ic*ic*(1/8-m*costheta/3/pi);
SPloss_igbt = fs*(Eon_igbt+Eoff_igbt);
SPloss_diode = fs*Erec_diode;

CPloss_igbt = CPloss_igbt*parallel;
CPloss_diode = CPloss_diode*parallel;
SPloss_igbt = SPloss_igbt*parallel;
SPloss_diode = SPloss_diode*parallel;

if ic == 0
    SPloss_igbt = 0;
    SPloss_diode = 0;
end
end

== matlab function BEV_Laengsdynamikmodell_v2/Voltage_quick_fix/MATLAB Function ==
  data: y output
function y = fcn()
y = 0;
coder.extrinsic('evalin');

y = evalin('base', 'acc_cycle_flag');

end

== matlab function BEV_Laengsdynamikmodell_v2/Current_fix/MATLAB Function ==
  data: y output
function y = fcn()
y = 0;
coder.extrinsic('evalin');

y = evalin('base', 'acc_cycle_flag');

end

== matlab function BEV_Laengsdynamikmodell_v2/Variant Subsystem Battery/Battery Analytic (RC3)/Battery/battery voltage checker - 50%/MATLAB Function2 ==
  data: u input; y output; d input; st output; z input
function [y,st]= fcn(u, d, z)

y = u;
st = 0;

if u == 1 && d == 0
    if z == 1
    warning("Battery: Voltage went below 50%")
    else
        warning("Battery: Stopping simulation as voltage went below 50% in Main Driving Cycle")
        st = 1;
    end
end

== matlab function BEV_Laengsdynamikmodell_v2/Variant Subsystem Battery/Battery Analytic (RC3)/Battery/MATLAB Function3 ==
  settings: updateMethod=DISCRETE
  data: car_current input; parallel_cells input; V0_matCell input; iCell output; numCyclesCell output; socCell output; socParallelAssembly output; temperatureCell output; vCell output; vParallelAssembly output; R0_matCell input; AH_Cell input; thermal_massCell input; CoolantResistance input; AmbientResistance input; InitialSOC input; T_battery input; SOC_vecCell input; T_vecCell input; CellBalancingClosedResistance input; T_coolant input; T_ambient input; R1_matCell input; R2_matCell input; R3_matCell input; tau1_matCell input; tau2_matCell input; tau3_matCell input; time input; P_bat_loss output; simulation_charge_dynamics input
function [iCell, numCyclesCell, socCell, socParallelAssembly, temperatureCell, vCell, vParallelAssembly, P_bat_loss] = fcn(car_current, parallel_cells, V0_matCell, R0_matCell, AH_Cell, ...
    thermal_massCell, CoolantResistance, AmbientResistance, InitialSOC, T_battery, SOC_vecCell, T_vecCell, CellBalancingClosedResistance, T_coolant, T_ambient, R1_matCell, R2_matCell, R3_matCell, tau1_matCell, tau2_matCell, tau3_matCell, time, simulation_charge_dynamics)
    
 
    % Initialize Parameters
    dt = 1;  % Time step in seconds
    T_target_inital = 298.15;
    alpha = 1.25e-4;
    T_target = T_target_inital + alpha * time;  % Target temperature in K (e.g., 25°C)
    K_p = 0.1;  % Proportional gain for PI controller
    K_i = 0.01;  % Integral gain for PI control
    persistent numCyclesCell_previous soc_previous T_battery_previous integral_error;
    persistent v_dynamic1_prev v_dynamic2_prev v_dynamic3_prev;

    if isempty(soc_previous)
        soc_previous = InitialSOC;  % Set initial state of charge
        numCyclesCell_previous = 0;  % Initial number of cycles
        T_battery_previous = T_battery;  % Initial battery temperature
        integral_error = 0;  % Initialize integral term for PI control
        v_dynamic1_prev = 0;  % Initialize dynamic voltage components
        v_dynamic2_prev = 0;
        v_dynamic3_prev = 0;
    end

    % Battery Current (car_current as input)
    iCell = car_current / parallel_cells;  % Current flowing through each cell

    % Update State of Charge using Coulomb counting
    if iCell ~= 0
        socCell = soc_previous - (-iCell * dt / (3600 * AH_Cell));  % Updated SOC
    else
        socCell = soc_previous;  % No change if no current
    end
    socCell = max(0, min(socCell, 1));  % Ensure SOC stays within valid range [0, 1]

    % Update cycle count
    delta_soc = soc_previous - socCell;
    numCyclesIncrement = max(0, delta_soc);
    numCyclesCell_previous = numCyclesCell_previous + numCyclesIncrement;
    numCyclesCell = numCyclesCell_previous;
    socParallelAssembly = socCell;

    % Heat Transfer Calculations
    Q_ambient = (T_battery_previous - T_ambient) / AmbientResistance;

    % PI control for dynamic mass flow rate
    error = T_battery_previous - T_target;
    integral_error = integral_error + error * dt;
    mass_dot = max(0, K_p * error + K_i * integral_error);

    % Maximum mass flow rate limit
    Re = 2000; % Laminar flow
    mu = 8.9e-4; % Dynamic viscosity of water
    density = 1000; % Density of water
    D_h = 0.005; % Hydraulic diameter of pipe
    n = 4; % Number of channels
    A = (pi * n * D_h^2) / 4; % Cross-sectional area of channels
    cp = 4184; % Specific heat capacity of water
    v = (Re * mu) / (density * D_h); % Flow velocity of coolant
    
    mass_dot_max = density * A * v;
    mass_dot = min(mass_dot, mass_dot_max);

    Delta_T_initial = 0.03;   % Initial jump in temperature difference
    Delta_T_max = 0.04;       % Maximum temperature difference at steady state
    tau = 10;                 % Time constant, adjust based on system behavior
    beta = 4e-5;
    Temp_difference = Delta_T_initial + (Delta_T_max - Delta_T_initial) * (1 - exp(-time / tau)) + beta*time;

    Q_coolant = mass_dot * cp * Temp_difference;
    Q_total = Q_coolant + Q_ambient;

    % Iterative temperature calculation
    tolerance = 1e-3;
    max_iterations = 100;
    T_battery_new = T_battery_previous;
    iteration = 0;

    while true
        R0_interpolated = interp2(T_vecCell, SOC_vecCell, R0_matCell, T_battery_new, socCell, 'linear');
        R1_interpolated = interp2(T_vecCell, SOC_vecCell, R1_matCell, T_battery_new, socCell, 'linear');
        R2_interpolated = interp2(T_vecCell, SOC_vecCell, R2_matCell, T_battery_new, socCell, 'linear');
        tau1 = interp2(T_vecCell, SOC_vecCell, tau1_matCell, T_battery_new, socCell, 'linear');
        tau2 = interp2(T_vecCell, SOC_vecCell, tau2_matCell, T_battery_new, socCell, 'linear');
        
        R3_interpolated = interp2(T_vecCell, SOC_vecCell, R3_matCell, T_battery_new, socCell, 'linear');
        tau3 = interp2(T_vecCell, SOC_vecCell, tau3_matCell, T_battery_new, socCell, 'linear');
        
        if simulation_charge_dynamics == 2
            R3_interpolated = 0;
            tau3 = 1;
        end

        % Heat generated
        Q_generated = iCell^2 * (R0_interpolated + R1_interpolated + R2_interpolated + R3_interpolated);
        dT_battery_dt = (Q_generated - Q_total) / thermal_massCell;
        T_battery_new_next = T_battery_previous + dT_battery_dt * dt;

        % Check convergence
        if abs(T_battery_new_next - T_battery_new) < tolerance
            break;
        end
        T_battery_new = T_battery_new_next;
        iteration = iteration + 1;

        if iteration >= max_iterations
            warning('Temperature calculation did not converge within max iterations');
            break;
        end
    end

    T_battery_new = T_battery_new_next;
    temperatureCell = T_battery_new;

    % Interpolated OCV
    V0_interpolated = interp2(T_vecCell, SOC_vecCell, V0_matCell, T_battery_new, socCell, 'linear');

    % Dynamic voltage drop (polarization effects) with updated time-stepping
    v_dynamic1 = v_dynamic1_prev + (-iCell * R1_interpolated - v_dynamic1_prev) * (1 - exp(-dt / tau1));
    v_dynamic2 = v_dynamic2_prev + (-iCell * R2_interpolated - v_dynamic2_prev) * (1 - exp(-dt / tau2));
    v_dynamic3 = v_dynamic3_prev + (-iCell * R3_interpolated - v_dynamic3_prev) * (1 - exp(-dt / tau3));

    % Total dynamic voltage drop
    v_dynamic = v_dynamic1 + v_dynamic2 + v_dynamic3;

    % Calculate vCell including dynamic effects
    vCell = V0_interpolated - (-iCell * R0_interpolated) - v_dynamic;

    % Voltage for Parallel Assembly
    vParallelAssembly = vCell;

    % Update previous state variables for the next time step
    soc_previous = socCell;
    T_battery_previous = T_battery_new;
    v_dynamic1_prev = v_dynamic1;
    v_dynamic2_prev = v_dynamic2;
    v_dynamic3_prev = v_dynamic3;

    % Ohmic losses
    Q_ohmic = Q_generated;
    % Dynamic voltage losses
    P_polarization = iCell * (v_dynamic1 + v_dynamic2 + v_dynamic3);
    % Total losses
    Q_total_loss = Q_ohmic + P_polarization;
    
    P_bat_loss = Q_total_loss;
    
    if isnan(P_bat_loss)
        warning('P_bat_loss is NaN.');
        P_bat_loss =0;
    end
end

== matlab function BEV_Laengsdynamikmodell_v2/Variant Subsystem Inverter/Inverter Analytic/Variant Subsystem/IM_Inverter_IGBT_Analytic/MATLAB Function3 ==
  data: u output; T_m input; i output; usq input; usd input; costheta output; n input
function [u, i, costheta] = fcn(T_m, usq, usd, n)

   Lm = 4.5e-4;
   Lr =  0.01571 + Lm;
   p = 3;
   T_e = T_m/p;
   
   if T_m >=0
       id = -sqrt((2*T_e/p*Lr)/(3*p*Lm^2));
   else
       id = sqrt((-2*T_e/p*Lr)/(3*p*Lm^2));
   end
   iq = id;
   i = sqrt(id^2 + iq^2)/2;
   u = sqrt(usq*usq+usd*usd);
   costheta = (usd*id+usq*iq)/u/i;

   if isnan(costheta)
       costheta = 1;
   end

   if n < 0.1
       u = 0;
       i = 0;
       costheta = 1;
   end

end

== matlab function BEV_Laengsdynamikmodell_v2/Variant Subsystem Inverter/Inverter Analytic/Variant Subsystem/IM_Inverter_SiC-MOSFET_Analytic/MATLAB Function ==
  data: t input; udc input; w_mech input; u_sq output; u_sd output
function [u_sq, u_sd] = fcn(t, udc, w_mech)
    
    p = 3; %pole pairs
    
    V_line = udc/2;
    V_phase = V_line/sqrt(3);
    w_elect = p * w_mech;
    
    V_a = V_phase * sin(w_elect * t);
    V_b = V_phase * sin(w_elect * t - 2*pi/3);
    V_c = V_phase * sin(w_elect * t + 2*pi/3);

    % Transformation from abc to dq reference frame
    % Assuming stator flux-oriented control with d-axis aligned with rotor flux
    theta_e = w_elect * t; % Electrical angle
    
    % Clarke transformation to alpha-beta reference frame
    V_alpha = (2/3) * (V_a - 0.5 * (V_b + V_c));
    V_beta = (2/3) * ((sqrt(3)/2) * (V_b - V_c));
    
    % Park transformation to d-q reference frame
    u_sd = V_alpha * cos(theta_e) + V_beta * sin(theta_e);
    u_sq = -V_alpha * sin(theta_e) + V_beta * cos(theta_e);

end

== matlab function BEV_Laengsdynamikmodell_v2/Variant Subsystem Gearbox/Gearbox Lookup-Table/Oil Temp/MATLAB Function ==
  data: t input; P_V input; T output
function T = fcn(t, P_V)

coder.extrinsic('evalin');

% Calculate lubricant temperature
ambient_temp = 0;
ambient_temp = evalin('base', 'config_vehicle.ambient_temp');
% 
% if t < (ambient_temp - 273)
%     T = (ambient_temp - 273);
% elseif t <= 70 %Aufwärmphase mit Umgebung < t < 70°C
%     T = abs(P) * 0.0003 + rpm * 0.00004 + t; %Leistungsabhängiger und drehzahlabhängiger Energieeintrag (Temperaturanstieg)
% else %Temperatur t > 70°C -> Wärmeabgabe ~ delta_t und ~ delta_t^2 (mit delta_t = t_gearbox - t_ambient)
%     T = abs(P) * 0.0003 + rpm * 0.00004 + t - (t - ambient_temp + 273) * 0.0002 - (t - ambient_temp + 273)^2 * 0.0000022;
% end

if t < (ambient_temp - 273)
    T = (ambient_temp - 273);
elseif t <= 80 %Aufwärmphase mit Umgebung < t < 70°C
    T =0.000055*P_V + t - (t - ambient_temp + 273) * 0.0003; %Leistungsabhängiger und drehzahlabhängiger Energieeintrag (Temperaturanstieg)
else %Temperatur t > 70°C -> Wärmeabgabe ~ delta_t und ~ delta_t^2 (mit delta_t = t_gearbox - t_ambient)
    T = 0.000088*P_V + t - (t - ambient_temp + 273) * 0.0010 - (t - ambient_temp + 273)^2 * 0.000012;
end

end

== matlab function BEV_Laengsdynamikmodell_v2/Variant Subsystem Inverter/Inverter Analytic/Variant Subsystem/PMSM_Inverter_SiC-MOSFET_Analytic/MATLAB Function ==
  data: u input; y output
function y = fcn(u)
    if isnan(u)
        warning('P_inveter_loss is NaN. ');
  
    end

    y=u;

== matlab function BEV_Laengsdynamikmodell_v2/MATLAB Function ==
  data: u input; y output
function y = fcn(u)
    if isnan(u)
        warning('P_inveter_loss is NaN. ');

    end
    y=u;
